simulink model "OMSv1_5_lfd"  (Simulink 7.0)
settings: Solver=ode4  SolverMode=SingleTasking  StartTime=0.0  StopTime=4  FixedStep=0.001  MaxStep=0.001  RelTol=1e-3  AbsTol=1e-3
undefined symbols (not defined in the file): alexlaw, bs_onoff, bs_scale, bsfsacrit, bsfsvcrit, cnsgain, fs_onoff, fs_scale, fsdelaycalc, ltdrk, mdlparamlist, phasicgain, pmcgain, pmctau2, pmctau3, saccsw, spgain, tonicgain, tvrD, tvrN
(part 7 of 10)

== system OMSv1_5_lfd/OMS v1.4  12/31/07/IM CN-LMLN/Sampled Target Reconstruction/SampHold?/Sign ==
  in_1 : Inport  OutDataType=sfix(16)  OutScaling=2^0
  Constant : Constant  Value=0  OutDataType=sfix(16)  OutScaling=2^0
  Relational Operator : RelationalOperator  Operator=>  InputSameDT=on
  Relational Operator1 : RelationalOperator  Operator=<  InputSameDT=on
  Sum : Sum  Inputs=+-  OutDataType=sfix(16)  OutScaling=2^0  SaturateOnIntegerOverflow=on  InputSameDT=on
  out_1 : Outport  OutDataType=sfix(16)  OutScaling=2^0  InitialOutput=0
  wires:
  Sum/1 -> out_1/1
  Relational Operator/1 -> Sum/1
  Relational Operator1/1 -> Sum/2
  Constant/1 -> Relational Operator1/2, Relational Operator/2
  in_1/1 -> Relational Operator/1, Relational Operator1/1

== system OMSv1_5_lfd/OMS v1.4  12/31/07/IM CN-LMLN/Sampled Target Reconstruction/leading edge detect1/Sign ==
  in_1 : Inport  OutDataType=sfix(16)  OutScaling=2^0
  Constant : Constant  Value=0  OutDataType=sfix(16)  OutScaling=2^0
  Relational Operator : RelationalOperator  Operator=>  InputSameDT=on
  Relational Operator1 : RelationalOperator  Operator=<  InputSameDT=on
  Sum : Sum  Inputs=+-  OutDataType=sfix(16)  OutScaling=2^0  SaturateOnIntegerOverflow=on  InputSameDT=on
  out_1 : Outport  OutDataType=sfix(16)  OutScaling=2^0  InitialOutput=0
  wires:
  in_1/1 -> Relational Operator1/1, Relational Operator/1
  Constant/1 -> Relational Operator/2, Relational Operator1/2
  Relational Operator1/1 -> Sum/2
  Relational Operator/1 -> Sum/1
  Sum/1 -> out_1/1

== system OMSv1_5_lfd/OMS v1.4  12/31/07/IM CN-LMLN/Sampled Target Reconstruction/leading edge detect2/Sign ==
  in_1 : Inport  OutDataType=sfix(16)  OutScaling=2^0
  Constant : Constant  Value=0  OutDataType=sfix(16)  OutScaling=2^0
  Relational Operator : RelationalOperator  Operator=>  InputSameDT=on
  Relational Operator1 : RelationalOperator  Operator=<  InputSameDT=on
  Sum : Sum  Inputs=+-  OutDataType=sfix(16)  OutScaling=2^0  SaturateOnIntegerOverflow=on  InputSameDT=on
  out_1 : Outport  OutDataType=sfix(16)  OutScaling=2^0  InitialOutput=0
  wires:
  Sum/1 -> out_1/1
  Relational Operator/1 -> Sum/1
  Relational Operator1/1 -> Sum/2
  Constant/1 -> Relational Operator1/2, Relational Operator/2
  in_1/1 -> Relational Operator/1, Relational Operator1/1

== system OMSv1_5_lfd/OMS v1.4  12/31/07/IM CN-LMLN/Sampled Target Reconstruction/prolong/Latch1 ==
  in_1 : Inport  OutDataType=sfix(16)  OutScaling=2^0
  in_2 : Inport  Port=2  OutDataType=sfix(16)  OutScaling=2^0
  Demux : Demux  Outputs=2
  Logic : CombinatorialLogic  TruthTable=[0 1;0 1;1 0;0 1;1 0;0 1;1 0;1 0]
  Memory : Memory  Orientation=left  X0=ini
  Mux : Mux  Inputs=3
  out_1 : Outport  OutDataType=sfix(16)  OutScaling=2^0  InitialOutput=0
  out_2 : Outport  Port=2  OutDataType=sfix(16)  OutScaling=2^0  InitialOutput=0
  wires:
  in_2/1 -> Mux/3
  in_1/1 -> Mux/2
  Memory/1 -> Mux/1
  Demux/1 -> Memory/1, out_1/1
  Mux/1 -> Logic/1
  Logic/1 -> Demux/1
  Demux/2 -> out_2/1

== system OMSv1_5_lfd/OMS v1.4  12/31/07/IM CN-LMLN/Sampled Target Reconstruction/prolong/SampHold?2 ==
  note: When "S/H?" is LOW, then "Input" is switched directly to the
      | output ("sample").  When "S/H?" is HIGH, the current output is
      | maintained ("hold").
  Input : Inport  OutDataType=sfix(16)  OutScaling=2^0
  S/H? : Inport  Port=2  OutDataType=sfix(16)  OutScaling=2^0
  Memory : Memory  Orientation=left
  Sign : Subsystem
      mask Type: Sign
      mask Description: y = sign(x)
      mask Help: Sign Function:\n\t\t\ty = 1 if x > 0\n\t\t\ty = 0 if x = 0\n\t\t\ty = -1 if x < 0
      mask Display: plot(-50,-50,50,50,[-50,50],[0,0],[0,0],[-50,50],[-40,0],[-30,-30],[0,40],[30,30])
  Switch2 : Switch  Threshold=0.5  SaturateOnIntegerOverflow=on  InputSameDT=on
  output : Outport  OutDataType=sfix(16)  OutScaling=2^0  InitialOutput=0
  wires:
  S/H?/1 -> Sign/1(in_1)
  Sign/1(out_1) -> Switch2/2
  Input/1 -> Switch2/3
  Switch2/1 -> Memory/1, output/1
  Memory/1 -> Switch2/1

== system OMSv1_5_lfd/OMS v1.4  12/31/07/IM CN-LMLN/Sampled Target Reconstruction/prolong/leading edge detect ==
  note: leading edge detection
  in_1 : Inport  OutDataType=sfix(16)  OutScaling=2^0
  Abs : Abs  SaturateOnIntegerOverflow=on
  Derivative : Derivative
  Relational Operator : RelationalOperator  Operator===  InputSameDT=on
  Sign : Subsystem
      mask Type: Sign
      mask Description: y = sign(x)
      mask Help: Sign Function:\n\t\t\ty = 1 if x > 0\n\t\t\ty = 0 if x = 0\n\t\t\ty = -1 if x < 0
      mask Display: plot(-50,-50,50,50,[-50,50],[0,0],[0,0],[-50,50],[-40,0],[-30,-30],[0,40],[30,30])
  Threshold 1 : Constant  OutDataType=sfix(16)  OutScaling=2^0
  out_1 : Outport  OutDataType=sfix(16)  OutScaling=2^0  InitialOutput=0
  wires:
  in_1/1 -> Abs/1
  Relational Operator/1 -> out_1/1
  Threshold 1/1 -> Relational Operator/2
  Sign/1(out_1) -> Relational Operator/1
  Derivative/1 -> Sign/1(in_1)
  Abs/1 -> Derivative/1

== system OMSv1_5_lfd/OMS v1.4  12/31/07/IM CN-LMLN/Sampled Target Reconstruction/prolong/trailing edge detect ==
  note: It is also possible to remove the SIGNUM function
      | and the '==', and replace them with a simple
      | switch with a threshold of (say) 150 or so.
  note: trailing edge detection
  in_1 : Inport  OutDataType=sfix(16)  OutScaling=2^0
  Abs : Abs  SaturateOnIntegerOverflow=on
  Derivative : Derivative
  Relational Operator : RelationalOperator  Operator===  InputSameDT=on
  Sign : Subsystem
      mask Type: Sign
      mask Description: y = sign(x)
      mask Help: Sign Function:\n\t\t\ty = 1 if x > 0\n\t\t\ty = 0 if x = 0\n\t\t\ty = -1 if x < 0
      mask Display: plot(-50,-50,50,50,[-50,50],[0,0],[0,0],[-50,50],[-40,0],[-30,-30],[0,40],[30,30])
  Threshold 1 : Constant  Value=-1  OutDataType=sfix(16)  OutScaling=2^0
  out_1 : Outport  OutDataType=sfix(16)  OutScaling=2^0  InitialOutput=0
  wires:
  Abs/1 -> Derivative/1
  Derivative/1 -> Sign/1(in_1)
  Sign/1(out_1) -> Relational Operator/1
  Threshold 1/1 -> Relational Operator/2
  Relational Operator/1 -> out_1/1
  in_1/1 -> Abs/1

== system OMSv1_5_lfd/OMS v1.4  12/31/07/IM CN-LMLN/Sampled Target Reconstruction/prolong1/Latch1 ==
  in_1 : Inport  OutDataType=sfix(16)  OutScaling=2^0
  in_2 : Inport  Port=2  OutDataType=sfix(16)  OutScaling=2^0
  Demux : Demux  Outputs=2
  Logic : CombinatorialLogic  TruthTable=[0 1;0 1;1 0;0 1;1 0;0 1;1 0;1 0]
  Memory : Memory  Orientation=left  X0=ini
  Mux : Mux  Inputs=3
  out_1 : Outport  OutDataType=sfix(16)  OutScaling=2^0  InitialOutput=0
  out_2 : Outport  Port=2  OutDataType=sfix(16)  OutScaling=2^0  InitialOutput=0
  wires:
  Demux/2 -> out_2/1
  Logic/1 -> Demux/1
  Mux/1 -> Logic/1
  Demux/1 -> out_1/1, Memory/1
  Memory/1 -> Mux/1
  in_1/1 -> Mux/2
  in_2/1 -> Mux/3

== system OMSv1_5_lfd/OMS v1.4  12/31/07/IM CN-LMLN/Sampled Target Reconstruction/prolong1/SampHold?2 ==
  note: When "S/H?" is LOW, then "Input" is switched directly to the
      | output ("sample").  When "S/H?" is HIGH, the current output is
      | maintained ("hold").
  Input : Inport  OutDataType=sfix(16)  OutScaling=2^0
  S/H? : Inport  Port=2  OutDataType=sfix(16)  OutScaling=2^0
  Memory : Memory  Orientation=left
  Sign : Subsystem
      mask Type: Sign
      mask Description: y = sign(x)
      mask Help: Sign Function:\n\t\t\ty = 1 if x > 0\n\t\t\ty = 0 if x = 0\n\t\t\ty = -1 if x < 0
      mask Display: plot(-50,-50,50,50,[-50,50],[0,0],[0,0],[-50,50],[-40,0],[-30,-30],[0,40],[30,30])
  Switch2 : Switch  Threshold=0.5  SaturateOnIntegerOverflow=on  InputSameDT=on
  output : Outport  OutDataType=sfix(16)  OutScaling=2^0  InitialOutput=0
  wires:
  Memory/1 -> Switch2/1
  Switch2/1 -> output/1, Memory/1
  Input/1 -> Switch2/3
  Sign/1(out_1) -> Switch2/2
  S/H?/1 -> Sign/1(in_1)

== system OMSv1_5_lfd/OMS v1.4  12/31/07/IM CN-LMLN/Sampled Target Reconstruction/prolong1/leading edge detect ==
  note: leading edge detection
  in_1 : Inport  OutDataType=sfix(16)  OutScaling=2^0
  Abs : Abs  SaturateOnIntegerOverflow=on
  Derivative : Derivative
  Relational Operator : RelationalOperator  Operator===  InputSameDT=on
  Sign : Subsystem
      mask Type: Sign
      mask Description: y = sign(x)
      mask Help: Sign Function:\n\t\t\ty = 1 if x > 0\n\t\t\ty = 0 if x = 0\n\t\t\ty = -1 if x < 0
      mask Display: plot(-50,-50,50,50,[-50,50],[0,0],[0,0],[-50,50],[-40,0],[-30,-30],[0,40],[30,30])
  Threshold 1 : Constant  OutDataType=sfix(16)  OutScaling=2^0
  out_1 : Outport  OutDataType=sfix(16)  OutScaling=2^0  InitialOutput=0
  wires:
  Abs/1 -> Derivative/1
  Derivative/1 -> Sign/1(in_1)
  Sign/1(out_1) -> Relational Operator/1
  Threshold 1/1 -> Relational Operator/2
  Relational Operator/1 -> out_1/1
  in_1/1 -> Abs/1

== system OMSv1_5_lfd/OMS v1.4  12/31/07/IM CN-LMLN/Sampled Target Reconstruction/prolong1/trailing edge detect ==
  note: trailing edge detection
  note: It is also possible to remove the SIGNUM function
      | and the '==', and replace them with a simple
      | switch with a threshold of (say) 150 or so.
  in_1 : Inport  OutDataType=sfix(16)  OutScaling=2^0
  Abs : Abs  SaturateOnIntegerOverflow=on
  Derivative : Derivative
  Relational Operator : RelationalOperator  Operator===  InputSameDT=on
  Sign : Subsystem
      mask Type: Sign
      mask Description: y = sign(x)
      mask Help: Sign Function:\n\t\t\ty = 1 if x > 0\n\t\t\ty = 0 if x = 0\n\t\t\ty = -1 if x < 0
      mask Display: plot(-50,-50,50,50,[-50,50],[0,0],[0,0],[-50,50],[-40,0],[-30,-30],[0,40],[30,30])
  Threshold 1 : Constant  Value=-1  OutDataType=sfix(16)  OutScaling=2^0
  out_1 : Outport  OutDataType=sfix(16)  OutScaling=2^0  InitialOutput=0
  wires:
  in_1/1 -> Abs/1
  Relational Operator/1 -> out_1/1
  Threshold 1/1 -> Relational Operator/2
  Sign/1(out_1) -> Relational Operator/1
  Derivative/1 -> Sign/1(in_1)
  Abs/1 -> Derivative/1

== system OMSv1_5_lfd/OMS v1.4  12/31/07/IM CN-LMLN/Sampled Target Reconstruction/prolong2/Latch1 ==
  in_1 : Inport  OutDataType=sfix(16)  OutScaling=2^0
  in_2 : Inport  Port=2  OutDataType=sfix(16)  OutScaling=2^0
  Demux : Demux  Outputs=2
  Logic : CombinatorialLogic  TruthTable=[0 1;0 1;1 0;0 1;1 0;0 1;1 0;1 0]
  Memory : Memory  Orientation=left  X0=ini
  Mux : Mux  Inputs=3
  out_1 : Outport  OutDataType=sfix(16)  OutScaling=2^0  InitialOutput=0
  out_2 : Outport  Port=2  OutDataType=sfix(16)  OutScaling=2^0  InitialOutput=0
  wires:
  in_2/1 -> Mux/3
  in_1/1 -> Mux/2
  Memory/1 -> Mux/1
  Demux/1 -> Memory/1, out_1/1
  Mux/1 -> Logic/1
  Logic/1 -> Demux/1
  Demux/2 -> out_2/1

== system OMSv1_5_lfd/OMS v1.4  12/31/07/IM CN-LMLN/Sampled Target Reconstruction/prolong2/SampHold?2 ==
  note: When "S/H?" is LOW, then "Input" is switched directly to the
      | output ("sample").  When "S/H?" is HIGH, the current output is
      | maintained ("hold").
  Input : Inport  OutDataType=sfix(16)  OutScaling=2^0
  S/H? : Inport  Port=2  OutDataType=sfix(16)  OutScaling=2^0
  Memory : Memory  Orientation=left
  Sign : Subsystem
      mask Type: Sign
      mask Description: y = sign(x)
      mask Help: Sign Function:\n\t\t\ty = 1 if x > 0\n\t\t\ty = 0 if x = 0\n\t\t\ty = -1 if x < 0
      mask Display: plot(-50,-50,50,50,[-50,50],[0,0],[0,0],[-50,50],[-40,0],[-30,-30],[0,40],[30,30])
  Switch2 : Switch  Threshold=0.5  SaturateOnIntegerOverflow=on  InputSameDT=on
  output : Outport  OutDataType=sfix(16)  OutScaling=2^0  InitialOutput=0
  wires:
  S/H?/1 -> Sign/1(in_1)
  Sign/1(out_1) -> Switch2/2
  Input/1 -> Switch2/3
  Switch2/1 -> Memory/1, output/1
  Memory/1 -> Switch2/1

== system OMSv1_5_lfd/OMS v1.4  12/31/07/IM CN-LMLN/Sampled Target Reconstruction/prolong2/leading edge detect ==
  note: leading edge detection
  in_1 : Inport  OutDataType=sfix(16)  OutScaling=2^0
  Abs : Abs  SaturateOnIntegerOverflow=on
  Derivative : Derivative
  Relational Operator : RelationalOperator  Operator===  InputSameDT=on
  Sign : Subsystem
      mask Type: Sign
      mask Description: y = sign(x)
      mask Help: Sign Function:\n\t\t\ty = 1 if x > 0\n\t\t\ty = 0 if x = 0\n\t\t\ty = -1 if x < 0
      mask Display: plot(-50,-50,50,50,[-50,50],[0,0],[0,0],[-50,50],[-40,0],[-30,-30],[0,40],[30,30])
  Threshold 1 : Constant  OutDataType=sfix(16)  OutScaling=2^0
  out_1 : Outport  OutDataType=sfix(16)  OutScaling=2^0  InitialOutput=0
  wires:
  in_1/1 -> Abs/1
  Relational Operator/1 -> out_1/1
  Threshold 1/1 -> Relational Operator/2
  Sign/1(out_1) -> Relational Operator/1
  Derivative/1 -> Sign/1(in_1)
  Abs/1 -> Derivative/1

== system OMSv1_5_lfd/OMS v1.4  12/31/07/IM CN-LMLN/Sampled Target Reconstruction/prolong2/trailing edge detect ==
  note: It is also possible to remove the SIGNUM function
      | and the '==', and replace them with a simple
      | switch with a threshold of (say) 150 or so.
  note: trailing edge detection
  in_1 : Inport  OutDataType=sfix(16)  OutScaling=2^0
  Abs : Abs  SaturateOnIntegerOverflow=on
  Derivative : Derivative
  Relational Operator : RelationalOperator  Operator===  InputSameDT=on
  Sign : Subsystem
      mask Type: Sign
      mask Description: y = sign(x)
      mask Help: Sign Function:\n\t\t\ty = 1 if x > 0\n\t\t\ty = 0 if x = 0\n\t\t\ty = -1 if x < 0
      mask Display: plot(-50,-50,50,50,[-50,50],[0,0],[0,0],[-50,50],[-40,0],[-30,-30],[0,40],[30,30])
  Threshold 1 : Constant  Value=-1  OutDataType=sfix(16)  OutScaling=2^0
  out_1 : Outport  OutDataType=sfix(16)  OutScaling=2^0  InitialOutput=0
  wires:
  Abs/1 -> Derivative/1
  Derivative/1 -> Sign/1(in_1)
  Sign/1(out_1) -> Relational Operator/1
  Threshold 1/1 -> Relational Operator/2
  Relational Operator/1 -> out_1/1
  in_1/1 -> Abs/1

== system OMSv1_5_lfd/OMS v1.4  12/31/07/IM CN-LMLN/Slip Velocity Reconstruction/SampHold?4/Sign ==
  in_1 : Inport  OutDataType=sfix(16)  OutScaling=2^0
  Constant : Constant  Value=0  OutDataType=sfix(16)  OutScaling=2^0
  Relational Operator : RelationalOperator  Operator=>  InputSameDT=on
  Relational Operator1 : RelationalOperator  Operator=<  InputSameDT=on
  Sum : Sum  Inputs=+-  OutDataType=sfix(16)  OutScaling=2^0  SaturateOnIntegerOverflow=on  InputSameDT=on
  out_1 : Outport  OutDataType=sfix(16)  OutScaling=2^0  InitialOutput=0
  wires:
  Sum/1 -> out_1/1
  Relational Operator/1 -> Sum/1
  Relational Operator1/1 -> Sum/2
  Constant/1 -> Relational Operator/2, Relational Operator1/2
  in_1/1 -> Relational Operator1/1, Relational Operator/1

== system OMSv1_5_lfd/OMS v1.4  12/31/07/PG w rNI2/PW funct/Input Switch/lead/trail edge det ==
  note: It is also possible to remove the SIGNUM function
      | and the '==', and replace them with a simple
      | switch with a threshold of (say) 150 or so.
  note: leading/trailing edge detection
  in_1 : Inport  OutDataType=sfix(16)  OutScaling=2^0
  Abs : Abs  SaturateOnIntegerOverflow=on
  Derivative : Derivative
  Relational Operator : RelationalOperator  Operator===  InputSameDT=on
  Sign : Subsystem
      mask Type: Sign
      mask Description: y = sign(x)
      mask Help: Sign Function:\n\t\t\ty = 1 if x > 0\n\t\t\ty = 0 if x = 0\n\t\t\ty = -1 if x < 0
      mask Display: plot(-50,-50,50,50,[-50,50],[0,0],[0,0],[-50,50],[-40,0],[-30,-30],[0,40],[30,30])
  Threshold 1 : Constant  OutDataType=sfix(16)  OutScaling=2^0
  out_1 : Outport  OutDataType=sfix(16)  OutScaling=2^0  InitialOutput=0
  wires:
  Abs/1 -> Relational Operator/1
  Sign/1(out_1) -> Abs/1
  Derivative/1 -> Sign/1(in_1)
  Threshold 1/1 -> Relational Operator/2
  Relational Operator/1 -> out_1/1
  in_1/1 -> Derivative/1

== system OMSv1_5_lfd/OMS v1.4  12/31/07/PG w rNI2/RefLatch (Default = 50ms)/trailing edge/S-R Flip-Flop ==
  in_1 : Inport  OutDataType=sfix(16)  OutScaling=2^0
  in_2 : Inport  Port=2  OutDataType=sfix(16)  OutScaling=2^0
  Demux : Demux  Outputs=2
  Logic : CombinatorialLogic  TruthTable=[0 1;0 1;1 0;0 1;1 0;0 1;1 0;1 0]
  Memory : Memory  Orientation=left  X0=ini
  Mux : Mux  Inputs=3
  out_1 : Outport  OutDataType=sfix(16)  OutScaling=2^0  InitialOutput=0
  out_2 : Outport  Port=2  OutDataType=sfix(16)  OutScaling=2^0  InitialOutput=0
  wires:
  in_2/1 -> Mux/3
  in_1/1 -> Mux/2
  Memory/1 -> Mux/1
  Demux/1 -> out_1/1, Memory/1
  Mux/1 -> Logic/1
  Logic/1 -> Demux/1
  Demux/2 -> out_2/1

== system OMSv1_5_lfd/OMS v1.4  12/31/07/PG w rNI2/RefLatch (Default = 50ms)/trailing edge/trailing edge det ==
  note: It is also possible to remove the SIGNUM function
      | and the '==', and replace them with a simple
      | switch with a threshold of (say) 150 or so.
  note: trailing edge detection
  in_1 : Inport  OutDataType=sfix(16)  OutScaling=2^0
  Abs : Abs  SaturateOnIntegerOverflow=on
  Derivative : Derivative
  Relational Operator : RelationalOperator  Operator===  InputSameDT=on
  Sign : Subsystem
      mask Type: Sign
      mask Description: y = sign(x)
      mask Help: Sign Function:\n\t\t\ty = 1 if x > 0\n\t\t\ty = 0 if x = 0\n\t\t\ty = -1 if x < 0
      mask Display: plot(-50,-50,50,50,[-50,50],[0,0],[0,0],[-50,50],[-40,0],[-30,-30],[0,40],[30,30])
  Threshold 1 : Constant  Value=-1  OutDataType=sfix(16)  OutScaling=2^0
  out_1 : Outport  OutDataType=sfix(16)  OutScaling=2^0  InitialOutput=0
  wires:
  Abs/1 -> Derivative/1
  Derivative/1 -> Sign/1(in_1)
  Sign/1(out_1) -> Relational Operator/1
  Threshold 1/1 -> Relational Operator/2
  Relational Operator/1 -> out_1/1
  in_1/1 -> Abs/1

== system OMSv1_5_lfd/OMS v1.4  12/31/07/PG w rNI2/RefLatch (Default = 50ms)/trailing edge/trailing edge det1 ==
  note: trailing edge detection
  note: It is also possible to remove the SIGNUM function
      | and the '==', and replace them with a simple
      | switch with a threshold of (say) 150 or so.
  in_1 : Inport  OutDataType=sfix(16)  OutScaling=2^0
  Abs : Abs  SaturateOnIntegerOverflow=on
  Derivative : Derivative
  Relational Operator : RelationalOperator  Operator===  InputSameDT=on
  Sign : Subsystem
      mask Type: Sign
      mask Description: y = sign(x)
      mask Help: Sign Function:\n\t\t\ty = 1 if x > 0\n\t\t\ty = 0 if x = 0\n\t\t\ty = -1 if x < 0
      mask Display: plot(-50,-50,50,50,[-50,50],[0,0],[0,0],[-50,50],[-40,0],[-30,-30],[0,40],[30,30])
  Threshold 1 : Constant  Value=-1  OutDataType=sfix(16)  OutScaling=2^0
  out_1 : Outport  OutDataType=sfix(16)  OutScaling=2^0  InitialOutput=0
  wires:
  in_1/1 -> Abs/1
  Relational Operator/1 -> out_1/1
  Threshold 1/1 -> Relational Operator/2
  Sign/1(out_1) -> Relational Operator/1
  Derivative/1 -> Sign/1(in_1)
  Abs/1 -> Derivative/1

== system OMSv1_5_lfd/OMS v1.4  12/31/07/oscillating PMC/NI Real3/Boolify/direction1 ==
  in_1 : Inport  OutDataType=sfix(16)  OutScaling=2^0
  Constant : Constant  Value=0  OutDataType=sfix(16)  OutScaling=2^0
  Relational Operator : RelationalOperator  Operator=>  InputSameDT=on
  Relational Operator1 : RelationalOperator  Operator=<  InputSameDT=on
  Sum : Sum  Inputs=+-  OutDataType=sfix(16)  OutScaling=2^0  SaturateOnIntegerOverflow=on  InputSameDT=on
  out_1 : Outport  OutDataType=sfix(16)  OutScaling=2^0  InitialOutput=0
  wires:
  in_1/1 -> Relational Operator/1, Relational Operator1/1
  Constant/1 -> Relational Operator1/2, Relational Operator/2
  Relational Operator1/1 -> Sum/2
  Relational Operator/1 -> Sum/1
  Sum/1 -> out_1/1

== system OMSv1_5_lfd/OMS v1.4  12/31/07/IM CN-LMLN/BS/FS Logic/BS Enable1/BS Timing/Latch1 ==
  in_1 : Inport  OutDataType=sfix(16)  OutScaling=2^0
  in_2 : Inport  Port=2  OutDataType=sfix(16)  OutScaling=2^0
  Demux : Demux  Outputs=2
  Logic : CombinatorialLogic  TruthTable=[0 1;0 1;1 0;0 1;1 0;0 1;1 0;1 0]
  Memory : Memory  Orientation=left  X0=ini
  Mux : Mux  Inputs=3
  out_1 : Outport  OutDataType=sfix(16)  OutScaling=2^0  InitialOutput=0
  out_2 : Outport  Port=2  OutDataType=sfix(16)  OutScaling=2^0  InitialOutput=0
  wires:
  in_2/1 -> Mux/3
  in_1/1 -> Mux/2
  Memory/1 -> Mux/1
  Demux/1 -> Memory/1, out_1/1
  Mux/1 -> Logic/1
  Logic/1 -> Demux/1
  Demux/2 -> out_2/1

== system OMSv1_5_lfd/OMS v1.4  12/31/07/IM CN-LMLN/BS/FS Logic/BS Enable1/BS Timing/event timer2 ==
  note: In 2) Subsequent events DO NOT reset the counter; it only resets when it
      | reaches zero
  note: 2) A new event (leading or trailing edge) is detected. -- Only case 1)
  note: 1) The count reaches its limit (set in "timer value") -- Both case 1) and 2)
  note: In 1), Any event (leading or trailing edge) will reset the counter so that it
      | counts down from the end trailing edge) of that event.
  note: It has TWO modes: 1) Event resettable and 2) Event Non-resettable
  note: The real trick here is understanding how to reload the countdown.
      | It resets if either of two conditions is met:
  note: The "OR" gate allows either of these conditions to reset the circuit.  The delay before the
      | "S" input of the flip-flop prevents both "S" and "R" from being set simultaneously, because
      | this would put the flip-flop in an undefined state.
  note: Therefore, an event first RESETS and then SETS the flip-flop.
  note: (Init input: 0)
  note: (FF init state: Q=0)
  note: (Init input: 0)
  note: This block is an RESETTABLE EVENT TIMER.  It outputs a spike of unit height xx milliseconds
      | (set by "timer value") after it detects an event ( i.e a TRAILING edge which represents the end of a
      |  saccadic pulse)
  note: Resettable
      | Event Timer
  _PG : Inport  OutDataType=sfix(16)  OutScaling=2^0
  _timer value (port) : Inport  Port=2  OutDataType=sfix(16)  OutScaling=2^0
  1 msec : TransportDelay  DelayTime=.001
  Clock : Clock
      settings: Decimation=10
  Latch1 : Subsystem  mask(Latch){@1=0}
      mask prompts: @1 "Initial State for Output "Q":"
      mask help: Latch
      mask init:
      | ini=(@1~=0);
      mask Help: Latches the S input.  When S (set) is one, the Q output  becomes one.  The output remains one until the R (reset) input becomes one, forcing the output to zero.  If both R and S are one, the latch will be in an undefined state.
      mask Display: disp('S   Q\n\nR  !Q')
  Logical Operator : Logic  Operator=OR  Inputs=3
  Logical Operator1 : Logic
  Logical Operator2 : Logic
  Relational Operator : RelationalOperator  InputSameDT=on
  SampHold?1 : Subsystem
      mask Display: disp('S&H\n(S=L)\n(H=H)')
  Sum : Sum  Inputs=+-  OutDataType=sfix(16)  OutScaling=2^0  SaturateOnIntegerOverflow=on  InputSameDT=on
  Terminator : Terminator
  event resettable? : Constant  Orientation=up  Value=0  OutDataType=sfix(16)  OutScaling=2^0
  leading edge detect : Subsystem
      mask Display: disp('Leading\nEdge Det')
  loop breaker : Memory  Orientation=left
  trailing edge detect : Subsystem
      mask Display: disp('Trailing\nEdge Det')
  out_1 : Outport  OutDataType=sfix(16)  OutScaling=2^0  InitialOutput=0
  wires:
  event resettable?/1 -> Logical Operator2/2, Logical Operator1/2
  leading edge detect/1(out_1) -> Logical Operator2/1
  Logical Operator2/1 -> Logical Operator/2
  trailing edge detect/1(out_1) -> Logical Operator1/1, 1 msec/1
  Logical Operator1/1 -> Logical Operator/1
  loop breaker/1 -> Logical Operator/3
  _PG/1 -> leading edge detect/1(in_1), trailing edge detect/1(in_1)
  Latch1/1(out_1) -> SampHold?1/2(S/H?)
  Relational Operator/1 -> out_1/1, loop breaker/1
  Sum/1 -> Relational Operator/1
  Clock/1 -> Sum/1, SampHold?1/1(Input)
  SampHold?1/1(output) -> Sum/2
  Logical Operator/1 -> Latch1/2(in_2)
  1 msec/1 -> Latch1/1(in_1)
  _timer value (port)/1 -> Relational Operator/2
  Latch1/2(out_2) -> Terminator/1

== system OMSv1_5_lfd/OMS v1.4  12/31/07/IM CN-LMLN/BS/FS Logic/BS Enable1/BS Timing/leading edge detect ==
  note: leading edge detection
  in_1 : Inport  OutDataType=sfix(16)  OutScaling=2^0
  Abs : Abs  SaturateOnIntegerOverflow=on
  Derivative : Derivative
  Relational Operator : RelationalOperator  Operator===  InputSameDT=on
  Sign : Subsystem
      mask Type: Sign
      mask Description: y = sign(x)
      mask Help: Sign Function:\n\t\t\ty = 1 if x > 0\n\t\t\ty = 0 if x = 0\n\t\t\ty = -1 if x < 0
      mask Display: plot(-50,-50,50,50,[-50,50],[0,0],[0,0],[-50,50],[-40,0],[-30,-30],[0,40],[30,30])
  Threshold 1 : Constant  OutDataType=sfix(16)  OutScaling=2^0
  out_1 : Outport  OutDataType=sfix(16)  OutScaling=2^0  InitialOutput=0
  wires:
  in_1/1 -> Abs/1
  Relational Operator/1 -> out_1/1
  Threshold 1/1 -> Relational Operator/2
  Sign/1(out_1) -> Relational Operator/1
  Derivative/1 -> Sign/1(in_1)
  Abs/1 -> Derivative/1

== system OMSv1_5_lfd/OMS v1.4  12/31/07/IM CN-LMLN/BS/FS Logic/FS Enable/FS Timing/Latch1 ==
  in_1 : Inport  OutDataType=sfix(16)  OutScaling=2^0
  in_2 : Inport  Port=2  OutDataType=sfix(16)  OutScaling=2^0
  Demux : Demux  Outputs=2
  Logic : CombinatorialLogic  TruthTable=[0 1;0 1;1 0;0 1;1 0;0 1;1 0;1 0]
  Memory : Memory  Orientation=left  X0=ini
  Mux : Mux  Inputs=3
  out_1 : Outport  OutDataType=sfix(16)  OutScaling=2^0  InitialOutput=0
  out_2 : Outport  Port=2  OutDataType=sfix(16)  OutScaling=2^0  InitialOutput=0
  wires:
  Demux/2 -> out_2/1
  Logic/1 -> Demux/1
  Mux/1 -> Logic/1
  Demux/1 -> out_1/1, Memory/1
  Memory/1 -> Mux/1
  in_1/1 -> Mux/2
  in_2/1 -> Mux/3

== system OMSv1_5_lfd/OMS v1.4  12/31/07/IM CN-LMLN/BS/FS Logic/FS Enable/FS Timing/event timer2 ==
  note: Resettable
      | Event Timer
  note: This block is an RESETTABLE EVENT TIMER.  It outputs a spike of unit height xx milliseconds
      | (set by "timer value") after it detects an event ( i.e a TRAILING edge which represents the end of a
      |  saccadic pulse)
  note: (Init input: 0)
  note: (FF init state: Q=0)
  note: (Init input: 0)
  note: Therefore, an event first RESETS and then SETS the flip-flop.
  note: The "OR" gate allows either of these conditions to reset the circuit.  The delay before the
      | "S" input of the flip-flop prevents both "S" and "R" from being set simultaneously, because
      | this would put the flip-flop in an undefined state.
  note: The real trick here is understanding how to reload the countdown.
      | It resets if either of two conditions is met:
  note: It has TWO modes: 1) Event resettable and 2) Event Non-resettable
  note: In 1), Any event (leading or trailing edge) will reset the counter so that it
      | counts down from the end trailing edge) of that event.
  note: 1) The count reaches its limit (set in "timer value") -- Both case 1) and 2)
  note: 2) A new event (leading or trailing edge) is detected. -- Only case 1)
  note: In 2) Subsequent events DO NOT reset the counter; it only resets when it
      | reaches zero
  _PG : Inport  OutDataType=sfix(16)  OutScaling=2^0
  _timer value (port) : Inport  Port=2  OutDataType=sfix(16)  OutScaling=2^0
  1 msec : TransportDelay  DelayTime=.001
  Clock : Clock
      settings: Decimation=10
  Latch1 : Subsystem  mask(Latch){@1=0}
      mask prompts: @1 "Initial State for Output "Q":"
      mask help: Latch
      mask init:
      | ini=(@1~=0);
      mask Help: Latches the S input.  When S (set) is one, the Q output  becomes one.  The output remains one until the R (reset) input becomes one, forcing the output to zero.  If both R and S are one, the latch will be in an undefined state.
      mask Display: disp('S   Q\n\nR  !Q')
  Logical Operator : Logic  Operator=OR  Inputs=3
  Logical Operator1 : Logic
  Logical Operator2 : Logic
  Relational Operator : RelationalOperator  InputSameDT=on
  SampHold?1 : Subsystem
      mask Display: disp('S&H\n(S=L)\n(H=H)')
  Sum : Sum  Inputs=+-  OutDataType=sfix(16)  OutScaling=2^0  SaturateOnIntegerOverflow=on  InputSameDT=on
  Terminator : Terminator
  event resettable? : Constant  Orientation=up  Value=0  OutDataType=sfix(16)  OutScaling=2^0
  leading edge detect : Subsystem
      mask Display: disp('Leading\nEdge Det')
  loop breaker : Memory  Orientation=left
  trailing edge detect : Subsystem
      mask Display: disp('Trailing\nEdge Det')
  out_1 : Outport  OutDataType=sfix(16)  OutScaling=2^0  InitialOutput=0
  wires:
  _timer value (port)/1 -> Relational Operator/2
  1 msec/1 -> Latch1/1(in_1)
  Logical Operator/1 -> Latch1/2(in_2)
  SampHold?1/1(output) -> Sum/2
  Clock/1 -> SampHold?1/1(Input), Sum/1
  Sum/1 -> Relational Operator/1
  Relational Operator/1 -> loop breaker/1, out_1/1
  Latch1/1(out_1) -> SampHold?1/2(S/H?)
  _PG/1 -> trailing edge detect/1(in_1), leading edge detect/1(in_1)
  loop breaker/1 -> Logical Operator/3
  Logical Operator1/1 -> Logical Operator/1
  trailing edge detect/1(out_1) -> 1 msec/1, Logical Operator1/1
  Logical Operator2/1 -> Logical Operator/2
  leading edge detect/1(out_1) -> Logical Operator2/1
  event resettable?/1 -> Logical Operator1/2, Logical Operator2/2
  Latch1/2(out_2) -> Terminator/1

== system OMSv1_5_lfd/OMS v1.4  12/31/07/IM CN-LMLN/BS/FS Logic/FS Enable/FS Timing/leading edge detect ==
  note: leading edge detection
  in_1 : Inport  OutDataType=sfix(16)  OutScaling=2^0
  Abs : Abs  SaturateOnIntegerOverflow=on
  Derivative : Derivative
  Relational Operator : RelationalOperator  Operator===  InputSameDT=on
  Sign : Subsystem
      mask Type: Sign
      mask Description: y = sign(x)
      mask Help: Sign Function:\n\t\t\ty = 1 if x > 0\n\t\t\ty = 0 if x = 0\n\t\t\ty = -1 if x < 0
      mask Display: plot(-50,-50,50,50,[-50,50],[0,0],[0,0],[-50,50],[-40,0],[-30,-30],[0,40],[30,30])
  Threshold 1 : Constant  OutDataType=sfix(16)  OutScaling=2^0
  out_1 : Outport  OutDataType=sfix(16)  OutScaling=2^0  InitialOutput=0
  wires:
  Abs/1 -> Derivative/1
  Derivative/1 -> Sign/1(in_1)
  Sign/1(out_1) -> Relational Operator/1
  Threshold 1/1 -> Relational Operator/2
  Relational Operator/1 -> out_1/1
  in_1/1 -> Abs/1

== system OMSv1_5_lfd/OMS v1.4  12/31/07/IM CN-LMLN/BS/FS Logic/FS Enable/SampHold?1/Sign ==
  in_1 : Inport  OutDataType=sfix(16)  OutScaling=2^0
  Constant : Constant  Value=0  OutDataType=sfix(16)  OutScaling=2^0
  Relational Operator : RelationalOperator  Operator=>  InputSameDT=on
  Relational Operator1 : RelationalOperator  Operator=<  InputSameDT=on
  Sum : Sum  Inputs=+-  OutDataType=sfix(16)  OutScaling=2^0  SaturateOnIntegerOverflow=on  InputSameDT=on
  out_1 : Outport  OutDataType=sfix(16)  OutScaling=2^0  InitialOutput=0
  wires:
  Sum/1 -> out_1/1
  Relational Operator/1 -> Sum/1
  Relational Operator1/1 -> Sum/2
  Constant/1 -> Relational Operator1/2, Relational Operator/2
  in_1/1 -> Relational Operator/1, Relational Operator1/1

== system OMSv1_5_lfd/OMS v1.4  12/31/07/IM CN-LMLN/BS/FS Logic/FS Enable/prolong/Latch1 ==
  in_1 : Inport  OutDataType=sfix(16)  OutScaling=2^0
  in_2 : Inport  Port=2  OutDataType=sfix(16)  OutScaling=2^0
  Demux : Demux  Outputs=2
  Logic : CombinatorialLogic  TruthTable=[0 1;0 1;1 0;0 1;1 0;0 1;1 0;1 0]
  Memory : Memory  Orientation=left  X0=ini
  Mux : Mux  Inputs=3
  out_1 : Outport  OutDataType=sfix(16)  OutScaling=2^0  InitialOutput=0
  out_2 : Outport  Port=2  OutDataType=sfix(16)  OutScaling=2^0  InitialOutput=0
  wires:
  in_2/1 -> Mux/3
  in_1/1 -> Mux/2
  Memory/1 -> Mux/1
  Demux/1 -> Memory/1, out_1/1
  Mux/1 -> Logic/1
  Logic/1 -> Demux/1
  Demux/2 -> out_2/1

== system OMSv1_5_lfd/OMS v1.4  12/31/07/IM CN-LMLN/BS/FS Logic/FS Enable/prolong/SampHold?2 ==
  note: When "S/H?" is LOW, then "Input" is switched directly to the
      | output ("sample").  When "S/H?" is HIGH, the current output is
      | maintained ("hold").
  Input : Inport  OutDataType=sfix(16)  OutScaling=2^0
  S/H? : Inport  Port=2  OutDataType=sfix(16)  OutScaling=2^0
  Memory : Memory  Orientation=left
  Sign : Subsystem
      mask Type: Sign
      mask Description: y = sign(x)
      mask Help: Sign Function:\n\t\t\ty = 1 if x > 0\n\t\t\ty = 0 if x = 0\n\t\t\ty = -1 if x < 0
      mask Display: plot(-50,-50,50,50,[-50,50],[0,0],[0,0],[-50,50],[-40,0],[-30,-30],[0,40],[30,30])
  Switch2 : Switch  Threshold=0.5  SaturateOnIntegerOverflow=on  InputSameDT=on
  output : Outport  OutDataType=sfix(16)  OutScaling=2^0  InitialOutput=0
  wires:
  S/H?/1 -> Sign/1(in_1)
  Sign/1(out_1) -> Switch2/2
  Input/1 -> Switch2/3
  Switch2/1 -> Memory/1, output/1
  Memory/1 -> Switch2/1

== system OMSv1_5_lfd/OMS v1.4  12/31/07/IM CN-LMLN/BS/FS Logic/FS Enable/prolong/leading edge detect ==
  note: leading edge detection
  in_1 : Inport  OutDataType=sfix(16)  OutScaling=2^0
  Abs : Abs  SaturateOnIntegerOverflow=on
  Derivative : Derivative
  Relational Operator : RelationalOperator  Operator===  InputSameDT=on
  Sign : Subsystem
      mask Type: Sign
      mask Description: y = sign(x)
      mask Help: Sign Function:\n\t\t\ty = 1 if x > 0\n\t\t\ty = 0 if x = 0\n\t\t\ty = -1 if x < 0
      mask Display: plot(-50,-50,50,50,[-50,50],[0,0],[0,0],[-50,50],[-40,0],[-30,-30],[0,40],[30,30])
  Threshold 1 : Constant  OutDataType=sfix(16)  OutScaling=2^0
  out_1 : Outport  OutDataType=sfix(16)  OutScaling=2^0  InitialOutput=0
  wires:
  in_1/1 -> Abs/1
  Relational Operator/1 -> out_1/1
  Threshold 1/1 -> Relational Operator/2
  Sign/1(out_1) -> Relational Operator/1
  Derivative/1 -> Sign/1(in_1)
  Abs/1 -> Derivative/1

== system OMSv1_5_lfd/OMS v1.4  12/31/07/IM CN-LMLN/BS/FS Logic/FS Enable/prolong/trailing edge detect ==
  note: It is also possible to remove the SIGNUM function
      | and the '==', and replace them with a simple
      | switch with a threshold of (say) 150 or so.
  note: trailing edge detection
  in_1 : Inport  OutDataType=sfix(16)  OutScaling=2^0
  Abs : Abs  SaturateOnIntegerOverflow=on
  Derivative : Derivative
  Relational Operator : RelationalOperator  Operator===  InputSameDT=on
  Sign : Subsystem
      mask Type: Sign
      mask Description: y = sign(x)
      mask Help: Sign Function:\n\t\t\ty = 1 if x > 0\n\t\t\ty = 0 if x = 0\n\t\t\ty = -1 if x < 0
      mask Display: plot(-50,-50,50,50,[-50,50],[0,0],[0,0],[-50,50],[-40,0],[-30,-30],[0,40],[30,30])
  Threshold 1 : Constant  Value=-1  OutDataType=sfix(16)  OutScaling=2^0
  out_1 : Outport  OutDataType=sfix(16)  OutScaling=2^0  InitialOutput=0
  wires:
  Abs/1 -> Derivative/1
  Derivative/1 -> Sign/1(in_1)
  Sign/1(out_1) -> Relational Operator/1
  Threshold 1/1 -> Relational Operator/2
  Relational Operator/1 -> out_1/1
  in_1/1 -> Abs/1

== system OMSv1_5_lfd/OMS v1.4  12/31/07/IM CN-LMLN/BS/FS Logic/FS or BS?/Boolify/direction1 ==
  in_1 : Inport  OutDataType=sfix(16)  OutScaling=2^0
  Constant : Constant  Value=0  OutDataType=sfix(16)  OutScaling=2^0
  Relational Operator : RelationalOperator  Operator=>  InputSameDT=on
  Relational Operator1 : RelationalOperator  Operator=<  InputSameDT=on
  Sum : Sum  Inputs=+-  OutDataType=sfix(16)  OutScaling=2^0  SaturateOnIntegerOverflow=on  InputSameDT=on
  out_1 : Outport  OutDataType=sfix(16)  OutScaling=2^0  InitialOutput=0
  wires:
  in_1/1 -> Relational Operator/1, Relational Operator1/1
  Constant/1 -> Relational Operator1/2, Relational Operator/2
  Relational Operator1/1 -> Sum/2
  Relational Operator/1 -> Sum/1
  Sum/1 -> out_1/1

== system OMSv1_5_lfd/OMS v1.4  12/31/07/IM CN-LMLN/BS/FS Logic/FS or BS?/SampHold?1/Sign ==
  in_1 : Inport  OutDataType=sfix(16)  OutScaling=2^0
  Constant : Constant  Value=0  OutDataType=sfix(16)  OutScaling=2^0
  Relational Operator : RelationalOperator  Operator=>  InputSameDT=on
  Relational Operator1 : RelationalOperator  Operator=<  InputSameDT=on
  Sum : Sum  Inputs=+-  OutDataType=sfix(16)  OutScaling=2^0  SaturateOnIntegerOverflow=on  InputSameDT=on
  out_1 : Outport  OutDataType=sfix(16)  OutScaling=2^0  InitialOutput=0
  wires:
  Sum/1 -> out_1/1
  Relational Operator/1 -> Sum/1
  Relational Operator1/1 -> Sum/2
  Constant/1 -> Relational Operator/2, Relational Operator1/2
  in_1/1 -> Relational Operator1/1, Relational Operator/1

== system OMSv1_5_lfd/OMS v1.4  12/31/07/IM CN-LMLN/BS/FS Logic/TCHNG Override/event timer2/Latch1 ==
  in_1 : Inport  OutDataType=sfix(16)  OutScaling=2^0
  in_2 : Inport  Port=2  OutDataType=sfix(16)  OutScaling=2^0
  Demux : Demux  Outputs=2
  Logic : CombinatorialLogic  TruthTable=[0 1;0 1;1 0;0 1;1 0;0 1;1 0;1 0]
  Memory : Memory  Orientation=left  X0=ini
  Mux : Mux  Inputs=3
  out_1 : Outport  OutDataType=sfix(16)  OutScaling=2^0  InitialOutput=0
  out_2 : Outport  Port=2  OutDataType=sfix(16)  OutScaling=2^0  InitialOutput=0
  wires:
  in_2/1 -> Mux/3
  in_1/1 -> Mux/2
  Memory/1 -> Mux/1
  Demux/1 -> Memory/1, out_1/1
  Mux/1 -> Logic/1
  Logic/1 -> Demux/1
  Demux/2 -> out_2/1

== system OMSv1_5_lfd/OMS v1.4  12/31/07/IM CN-LMLN/BS/FS Logic/TCHNG Override/event timer2/SampHold?1 ==
  note: When "S/H?" is LOW, then "Input" is switched directly to the
      | output ("sample").  When "S/H?" is HIGH, the current output is
      | maintained ("hold").
  Input : Inport  OutDataType=sfix(16)  OutScaling=2^0
  S/H? : Inport  Port=2  OutDataType=sfix(16)  OutScaling=2^0
  Memory : Memory  Orientation=left
  Sign : Subsystem
      mask Type: Sign
      mask Description: y = sign(x)
      mask Help: Sign Function:\n\t\t\ty = 1 if x > 0\n\t\t\ty = 0 if x = 0\n\t\t\ty = -1 if x < 0
      mask Display: plot(-50,-50,50,50,[-50,50],[0,0],[0,0],[-50,50],[-40,0],[-30,-30],[0,40],[30,30])
  Switch2 : Switch  Threshold=0.5  SaturateOnIntegerOverflow=on  InputSameDT=on
  output : Outport  OutDataType=sfix(16)  OutScaling=2^0  InitialOutput=0
  wires:
  Switch2/1 -> Memory/1, output/1
  Sign/1(out_1) -> Switch2/2
  S/H?/1 -> Sign/1(in_1)
  Memory/1 -> Switch2/1
  Input/1 -> Switch2/3

== system OMSv1_5_lfd/OMS v1.4  12/31/07/IM CN-LMLN/BS/FS Logic/TCHNG Override/event timer2/leading edge detect ==
  note: It is also possible to remove the SIGNUM function
      | and the '==', and replace them with a simple
      | switch with a threshold of (say) 150 or so.
  note: leading edge detection
  in_1 : Inport  OutDataType=sfix(16)  OutScaling=2^0
  Abs : Abs  SaturateOnIntegerOverflow=on
  Derivative : Derivative
  Relational Operator : RelationalOperator  Operator===  InputSameDT=on
  Sign : Subsystem
      mask Type: Sign
      mask Description: y = sign(x)
      mask Help: Sign Function:\n\t\t\ty = 1 if x > 0\n\t\t\ty = 0 if x = 0\n\t\t\ty = -1 if x < 0
      mask Display: plot(-50,-50,50,50,[-50,50],[0,0],[0,0],[-50,50],[-40,0],[-30,-30],[0,40],[30,30])
  Threshold 1 : Constant  OutDataType=sfix(16)  OutScaling=2^0
  out_1 : Outport  OutDataType=sfix(16)  OutScaling=2^0  InitialOutput=0
  wires:
  Abs/1 -> Derivative/1
  Derivative/1 -> Sign/1(in_1)
  Sign/1(out_1) -> Relational Operator/1
  Threshold 1/1 -> Relational Operator/2
  Relational Operator/1 -> out_1/1
  in_1/1 -> Abs/1

== system OMSv1_5_lfd/OMS v1.4  12/31/07/IM CN-LMLN/BS/FS Logic/TCHNG Override/event timer2/trailing edge detect ==
  note: trailing edge detection
  note: It is also possible to remove the SIGNUM function
      | and the '==', and replace them with a simple
      | switch with a threshold of (say) 150 or so.
  in_1 : Inport  OutDataType=sfix(16)  OutScaling=2^0
  Abs : Abs  SaturateOnIntegerOverflow=on
  Derivative : Derivative
  Relational Operator : RelationalOperator  Operator===  InputSameDT=on
  Sign : Subsystem
      mask Type: Sign
      mask Description: y = sign(x)
      mask Help: Sign Function:\n\t\t\ty = 1 if x > 0\n\t\t\ty = 0 if x = 0\n\t\t\ty = -1 if x < 0
      mask Display: plot(-50,-50,50,50,[-50,50],[0,0],[0,0],[-50,50],[-40,0],[-30,-30],[0,40],[30,30])
  Threshold 1 : Constant  Value=-1  OutDataType=sfix(16)  OutScaling=2^0
  out_1 : Outport  OutDataType=sfix(16)  OutScaling=2^0  InitialOutput=0
  wires:
  in_1/1 -> Abs/1
  Relational Operator/1 -> out_1/1
  Threshold 1/1 -> Relational Operator/2
  Sign/1(out_1) -> Relational Operator/1
  Derivative/1 -> Sign/1(in_1)
  Abs/1 -> Derivative/1

== system OMSv1_5_lfd/OMS v1.4  12/31/07/IM CN-LMLN/BS/FS Logic/TCHNG Override/leading edge detect/Sign ==
  in_1 : Inport  OutDataType=sfix(16)  OutScaling=2^0
  Constant : Constant  Value=0  OutDataType=sfix(16)  OutScaling=2^0
  Relational Operator : RelationalOperator  Operator=>  InputSameDT=on
  Relational Operator1 : RelationalOperator  Operator=<  InputSameDT=on
  Sum : Sum  Inputs=+-  OutDataType=sfix(16)  OutScaling=2^0  SaturateOnIntegerOverflow=on  InputSameDT=on
  out_1 : Outport  OutDataType=sfix(16)  OutScaling=2^0  InitialOutput=0
  wires:
  Sum/1 -> out_1/1
  Relational Operator/1 -> Sum/1
  Relational Operator1/1 -> Sum/2
  Constant/1 -> Relational Operator/2, Relational Operator1/2
  in_1/1 -> Relational Operator1/1, Relational Operator/1

== system OMSv1_5_lfd/OMS v1.4  12/31/07/IM CN-LMLN/BS/FS Logic/prolong/SampHold?2/Sign ==
  in_1 : Inport  OutDataType=sfix(16)  OutScaling=2^0
  Constant : Constant  Value=0  OutDataType=sfix(16)  OutScaling=2^0
  Relational Operator : RelationalOperator  Operator=>  InputSameDT=on
  Relational Operator1 : RelationalOperator  Operator=<  InputSameDT=on
  Sum : Sum  Inputs=+-  OutDataType=sfix(16)  OutScaling=2^0  SaturateOnIntegerOverflow=on  InputSameDT=on
  out_1 : Outport  OutDataType=sfix(16)  OutScaling=2^0  InitialOutput=0
  wires:
  in_1/1 -> Relational Operator/1, Relational Operator1/1
  Constant/1 -> Relational Operator1/2, Relational Operator/2
  Relational Operator1/1 -> Sum/2
  Relational Operator/1 -> Sum/1
  Sum/1 -> out_1/1

== system OMSv1_5_lfd/OMS v1.4  12/31/07/IM CN-LMLN/BS/FS Logic/prolong/leading edge detect/Sign ==
  in_1 : Inport  OutDataType=sfix(16)  OutScaling=2^0
  Constant : Constant  Value=0  OutDataType=sfix(16)  OutScaling=2^0
  Relational Operator : RelationalOperator  Operator=>  InputSameDT=on
  Relational Operator1 : RelationalOperator  Operator=<  InputSameDT=on
  Sum : Sum  Inputs=+-  OutDataType=sfix(16)  OutScaling=2^0  SaturateOnIntegerOverflow=on  InputSameDT=on
  out_1 : Outport  OutDataType=sfix(16)  OutScaling=2^0  InitialOutput=0
  wires:
  Sum/1 -> out_1/1
  Relational Operator/1 -> Sum/1
  Relational Operator1/1 -> Sum/2
  Constant/1 -> Relational Operator/2, Relational Operator1/2
  in_1/1 -> Relational Operator1/1, Relational Operator/1

== system OMSv1_5_lfd/OMS v1.4  12/31/07/IM CN-LMLN/BS/FS Logic/prolong/trailing edge detect/Sign ==
  in_1 : Inport  OutDataType=sfix(16)  OutScaling=2^0
  Constant : Constant  Value=0  OutDataType=sfix(16)  OutScaling=2^0
  Relational Operator : RelationalOperator  Operator=>  InputSameDT=on
  Relational Operator1 : RelationalOperator  Operator=<  InputSameDT=on
  Sum : Sum  Inputs=+-  OutDataType=sfix(16)  OutScaling=2^0  SaturateOnIntegerOverflow=on  InputSameDT=on
  out_1 : Outport  OutDataType=sfix(16)  OutScaling=2^0  InitialOutput=0
  wires:
  in_1/1 -> Relational Operator/1, Relational Operator1/1
  Constant/1 -> Relational Operator1/2, Relational Operator/2
  Relational Operator1/1 -> Sum/2
  Relational Operator/1 -> Sum/1
  Sum/1 -> out_1/1

== system OMSv1_5_lfd/OMS v1.4  12/31/07/IM CN-LMLN/MdlPlnt+2/OMN3/SampHold?/Sign ==
  in_1 : Inport  OutDataType=sfix(16)  OutScaling=2^0
  Constant : Constant  Value=0  OutDataType=sfix(16)  OutScaling=2^0
  Relational Operator : RelationalOperator  Operator=>  InputSameDT=on
  Relational Operator1 : RelationalOperator  Operator=<  InputSameDT=on
  Sum : Sum  Inputs=+-  OutDataType=sfix(16)  OutScaling=2^0  SaturateOnIntegerOverflow=on  InputSameDT=on
  out_1 : Outport  OutDataType=sfix(16)  OutScaling=2^0  InitialOutput=0
  wires:
  in_1/1 -> Relational Operator/1, Relational Operator1/1
  Constant/1 -> Relational Operator1/2, Relational Operator/2
  Relational Operator1/1 -> Sum/2
  Relational Operator/1 -> Sum/1
  Sum/1 -> out_1/1

== system OMSv1_5_lfd/OMS v1.4  12/31/07/IM CN-LMLN/Sacc Blank/event timer1/SampHold?1/Sign ==
  in_1 : Inport  OutDataType=sfix(16)  OutScaling=2^0
  Constant : Constant  Value=0  OutDataType=sfix(16)  OutScaling=2^0
  Relational Operator : RelationalOperator  Operator=>  InputSameDT=on
  Relational Operator1 : RelationalOperator  Operator=<  InputSameDT=on
  Sum : Sum  Inputs=+-  OutDataType=sfix(16)  OutScaling=2^0  SaturateOnIntegerOverflow=on  InputSameDT=on
  out_1 : Outport  OutDataType=sfix(16)  OutScaling=2^0  InitialOutput=0
  wires:
  in_1/1 -> Relational Operator/1, Relational Operator1/1
  Constant/1 -> Relational Operator1/2, Relational Operator/2
  Relational Operator1/1 -> Sum/2
  Relational Operator/1 -> Sum/1
  Sum/1 -> out_1/1

== system OMSv1_5_lfd/OMS v1.4  12/31/07/IM CN-LMLN/Sacc Blank/event timer1/leading edge detect/Sign ==
  in_1 : Inport  OutDataType=sfix(16)  OutScaling=2^0
  Constant : Constant  Value=0  OutDataType=sfix(16)  OutScaling=2^0
  Relational Operator : RelationalOperator  Operator=>  InputSameDT=on
  Relational Operator1 : RelationalOperator  Operator=<  InputSameDT=on
  Sum : Sum  Inputs=+-  OutDataType=sfix(16)  OutScaling=2^0  SaturateOnIntegerOverflow=on  InputSameDT=on
  out_1 : Outport  OutDataType=sfix(16)  OutScaling=2^0  InitialOutput=0
  wires:
  in_1/1 -> Relational Operator/1, Relational Operator1/1
  Constant/1 -> Relational Operator1/2, Relational Operator/2
  Relational Operator1/1 -> Sum/2
  Relational Operator/1 -> Sum/1
  Sum/1 -> out_1/1

== system OMSv1_5_lfd/OMS v1.4  12/31/07/IM CN-LMLN/Sacc Blank/event timer1/trailing edge detect/Sign ==
  in_1 : Inport  OutDataType=sfix(16)  OutScaling=2^0
  Constant : Constant  Value=0  OutDataType=sfix(16)  OutScaling=2^0
  Relational Operator : RelationalOperator  Operator=>  InputSameDT=on
  Relational Operator1 : RelationalOperator  Operator=<  InputSameDT=on
  Sum : Sum  Inputs=+-  OutDataType=sfix(16)  OutScaling=2^0  SaturateOnIntegerOverflow=on  InputSameDT=on
  out_1 : Outport  OutDataType=sfix(16)  OutScaling=2^0  InitialOutput=0
  wires:
  Sum/1 -> out_1/1
  Relational Operator/1 -> Sum/1
  Relational Operator1/1 -> Sum/2
  Constant/1 -> Relational Operator1/2, Relational Operator/2
  in_1/1 -> Relational Operator/1, Relational Operator1/1

== system OMSv1_5_lfd/OMS v1.4  12/31/07/IM CN-LMLN/Saccade Enable/Enable Control/2 ms/Latch1 ==
  in_1 : Inport  OutDataType=sfix(16)  OutScaling=2^0
  in_2 : Inport  Port=2  OutDataType=sfix(16)  OutScaling=2^0
  Demux : Demux  Outputs=2
  Logic : CombinatorialLogic  TruthTable=[0 1;0 1;1 0;0 1;1 0;0 1;1 0;1 0]
  Memory : Memory  Orientation=left  X0=ini
  Mux : Mux  Inputs=3
  out_1 : Outport  OutDataType=sfix(16)  OutScaling=2^0  InitialOutput=0
  out_2 : Outport  Port=2  OutDataType=sfix(16)  OutScaling=2^0  InitialOutput=0
  wires:
  Demux/2 -> out_2/1
  Logic/1 -> Demux/1
  Mux/1 -> Logic/1
  Demux/1 -> out_1/1, Memory/1
  Memory/1 -> Mux/1
  in_1/1 -> Mux/2
  in_2/1 -> Mux/3

== system OMSv1_5_lfd/OMS v1.4  12/31/07/IM CN-LMLN/Saccade Enable/Enable Control/2 ms/SampHold?2 ==
  note: When "S/H?" is LOW, then "Input" is switched directly to the
      | output ("sample").  When "S/H?" is HIGH, the current output is
      | maintained ("hold").
  Input : Inport  OutDataType=sfix(16)  OutScaling=2^0
  S/H? : Inport  Port=2  OutDataType=sfix(16)  OutScaling=2^0
  Memory : Memory  Orientation=left
  Sign : Subsystem
      mask Type: Sign
      mask Description: y = sign(x)
      mask Help: Sign Function:\n\t\t\ty = 1 if x > 0\n\t\t\ty = 0 if x = 0\n\t\t\ty = -1 if x < 0
      mask Display: plot(-50,-50,50,50,[-50,50],[0,0],[0,0],[-50,50],[-40,0],[-30,-30],[0,40],[30,30])
  Switch2 : Switch  Threshold=0.5  SaturateOnIntegerOverflow=on  InputSameDT=on
  output : Outport  OutDataType=sfix(16)  OutScaling=2^0  InitialOutput=0
  wires:
  Memory/1 -> Switch2/1
  Switch2/1 -> output/1, Memory/1
  Input/1 -> Switch2/3
  Sign/1(out_1) -> Switch2/2
  S/H?/1 -> Sign/1(in_1)

== system OMSv1_5_lfd/OMS v1.4  12/31/07/IM CN-LMLN/Saccade Enable/Enable Control/2 ms/leading edge detect ==
  note: leading edge detection
  in_1 : Inport  OutDataType=sfix(16)  OutScaling=2^0
  Abs : Abs  SaturateOnIntegerOverflow=on
  Derivative : Derivative
  Relational Operator : RelationalOperator  Operator===  InputSameDT=on
  Sign : Subsystem
      mask Type: Sign
      mask Description: y = sign(x)
      mask Help: Sign Function:\n\t\t\ty = 1 if x > 0\n\t\t\ty = 0 if x = 0\n\t\t\ty = -1 if x < 0
      mask Display: plot(-50,-50,50,50,[-50,50],[0,0],[0,0],[-50,50],[-40,0],[-30,-30],[0,40],[30,30])
  Threshold 1 : Constant  OutDataType=sfix(16)  OutScaling=2^0
  out_1 : Outport  OutDataType=sfix(16)  OutScaling=2^0  InitialOutput=0
  wires:
  Abs/1 -> Derivative/1
  Derivative/1 -> Sign/1(in_1)
  Sign/1(out_1) -> Relational Operator/1
  Threshold 1/1 -> Relational Operator/2
  Relational Operator/1 -> out_1/1
  in_1/1 -> Abs/1

== system OMSv1_5_lfd/OMS v1.4  12/31/07/IM CN-LMLN/Saccade Enable/Enable Control/2 ms/trailing edge detect ==
  note: trailing edge detection
  note: It is also possible to remove the SIGNUM function
      | and the '==', and replace them with a simple
      | switch with a threshold of (say) 150 or so.
  in_1 : Inport  OutDataType=sfix(16)  OutScaling=2^0
  Abs : Abs  SaturateOnIntegerOverflow=on
  Derivative : Derivative
  Relational Operator : RelationalOperator  Operator===  InputSameDT=on
  Sign : Subsystem
      mask Type: Sign
      mask Description: y = sign(x)
      mask Help: Sign Function:\n\t\t\ty = 1 if x > 0\n\t\t\ty = 0 if x = 0\n\t\t\ty = -1 if x < 0
      mask Display: plot(-50,-50,50,50,[-50,50],[0,0],[0,0],[-50,50],[-40,0],[-30,-30],[0,40],[30,30])
  Threshold 1 : Constant  Value=-1  OutDataType=sfix(16)  OutScaling=2^0
  out_1 : Outport  OutDataType=sfix(16)  OutScaling=2^0  InitialOutput=0
  wires:
  in_1/1 -> Abs/1
  Relational Operator/1 -> out_1/1
  Threshold 1/1 -> Relational Operator/2
  Sign/1(out_1) -> Relational Operator/1
  Derivative/1 -> Sign/1(in_1)
  Abs/1 -> Derivative/1
